simulink model "BatteryCtrl_V1"  (R2018a)
settings: Solver=VariableStepAuto  StartTime=0.0  StopTime=10.0  FixedStep=sampletime  RelTol=1e-3  EnableMultiTasking=on
PreLoadFcn:
  | BatteryCtrl_V1_BusInfo;
libraries: simulink x2
settings Model: Creator=IAEC nishito  LastModifiedBy=nishito
settings DataIOCC: LimitDataPoints=on  SaveFormat=Array  SignalLoggingSaveFormat=ModelDataLogs  SaveOutput=off
settings OptimizationCC: DefaultParameterBehavior=Inlined  ExpressionDepthLimit=2147483647  LifeSpan=inf
settings DebuggingCC: UnderspecifiedInitializationDetection=Classic  MergeDetectMultiDrivingBlocksExec=none  SolverPrmCheckMsg=warning  FcnCallInpInsideContextMsg=warning  StateNameClashWarn=warning  SFUnexpectedBacktrackingDiag=warning  SFNoUnconditionalDefaultTransitionDiag=warning  SFExecutionAtInitializationDiag=none
settings HardwareCC: ProdBitPerPointer=32  ProdBitPerSizeT=32  ProdBitPerPtrDiffT=32  ProdLargestAtomicFloat=None  ProdIntDivRoundTo=Undefined  ProdEndianess=Unspecified  ProdWordSize=32  ProdHWDeviceType=32-bit Generic
settings ModelReferenceCC: UpdateModelReferenceTargets=IfOutOfDate  PropagateSignalLabelsOutOfModel=off
settings CodeAppCC: StateflowObjectComments=on
settings GRTTargetCC: TargetLangStandard=C89/C90 (ANSI)  GeneratePreprocessorConditionals=Disable all  CombineOutputUpdateFcns=off  GRTInterface=on
settings ConfigComp: CovMetricSettings=dw  CovHtmlReporting=on  CovSaveCumulativeToWorkspaceVar=on  CovSaveSingleToWorkspaceVar=on  CovExternalEMLEnable=off  CovSFcnEnable=off

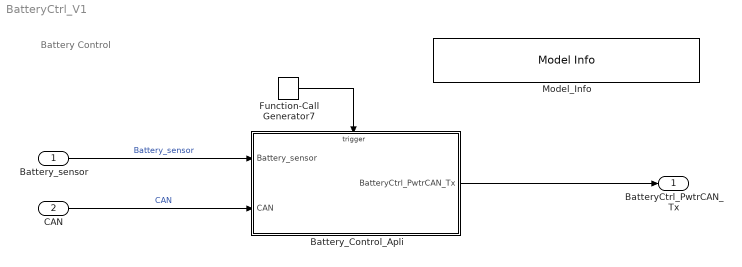
== system BatteryCtrl_V1 ==
  note: Battery Control
  Battery_sensor : Inport  OutDataTypeStr=Bus: Battery_sensor_Bus
      settings: AttributesFormatString=<%<OutDataTypeStr>>
  CAN : Inport  Port=2  OutDataTypeStr=Bus: CAN_Bus
      settings: AttributesFormatString=<%<OutDataTypeStr>>
  Battery_Control_Apli : Subsystem
  Function-Call Generator7 : simulink/Ports & Subsystems/Function-Call Generator  sample_time=0.05  numberOfIterations=1
      settings: AttributesFormatString=<sample_time=%<sample_time>>
  Model_Info : simulink/Model-Wide Utilities/Model Info  Frame=on  DisplayStringWithTags=|  HorizontalTextAlignment=Left  LeftAlignmentValue=0.02
      | Version  %<ModelVersion>
      | LastModifided by %<LastModifiedBy>  Date %<LastModificationDate>
      | Description  %<Description>
  BatteryCtrl_PwtrCAN_Tx : Outport  OutDataTypeStr=Bus: BatteryCtrl_PwtrCAN_Tx_Bus
      settings: AttributesFormatString=<%<OutDataTypeStr>>
  wires:
  Battery_Control_Apli/1(BatteryCtrl_PwtrCAN_Tx) -> BatteryCtrl_PwtrCAN_Tx/1
  CAN/1 -> Battery_Control_Apli/2(CAN)  "CAN"
  Battery_sensor/1 -> Battery_Control_Apli/1(Battery_sensor)  "Battery_sensor"
  Function-Call Generator7/1 -> Battery_Control_Apli/Trigger

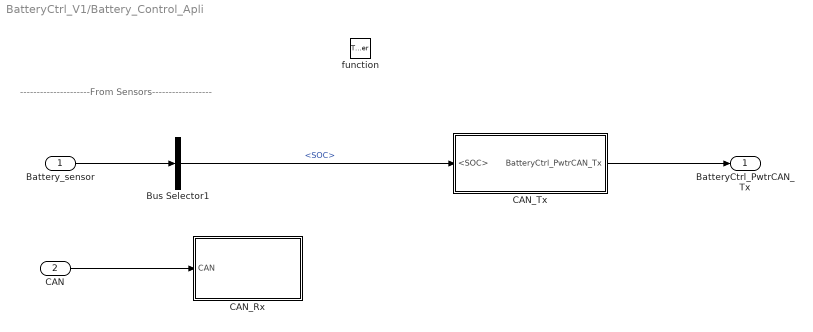
== system BatteryCtrl_V1/Battery_Control_Apli ==
  note: ---------------------From Sensors------------------
  Battery_sensor : Inport
  CAN : Inport  Port=2
  function : TriggerPort  TriggerType=function-call  VariantControl=Variant
  Bus Selector1 : BusSelector  OutputSignals=SOC
  CAN_Rx : Subsystem
  CAN_Tx : Subsystem
  BatteryCtrl_PwtrCAN_Tx : Outport
  wires:
  Battery_sensor/1 -> Bus Selector1/1
  Bus Selector1/1 -> CAN_Tx/1(<SOC>)  "<SOC>"
  CAN_Tx/1(BatteryCtrl_PwtrCAN_Tx) -> BatteryCtrl_PwtrCAN_Tx/1
  CAN/1 -> CAN_Rx/1(CAN)

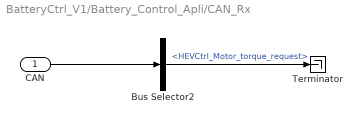
== system BatteryCtrl_V1/Battery_Control_Apli/CAN_Rx ==
  CAN : Inport
  Bus Selector2 : BusSelector  OutputSignals=PwtrCAN.HEV_Ctrl_PwtrCAN_Tx.HEVCtrl_Motor_torque_request
  Terminator : Terminator
  wires:
  CAN/1 -> Bus Selector2/1
  Bus Selector2/1 -> Terminator/1  "<HEVCtrl_Motor_torque_request>"

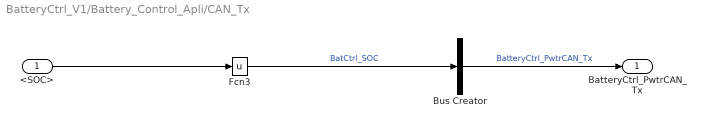
== system BatteryCtrl_V1/Battery_Control_Apli/CAN_Tx ==
  <SOC> : Inport
  Bus Creator : BusCreator  Inputs=1  OutDataTypeStr=Bus: BatteryCtrl_PwtrCAN_Tx_Bus
      settings: AttributesFormatString=<%<OutDataTypeStr>>
  Fcn3 : Fcn  Expr=u
  BatteryCtrl_PwtrCAN_Tx : Outport
  wires:
  Fcn3/1 -> Bus Creator/1  "BatCtrl_SOC"
  <SOC>/1 -> Fcn3/1
  Bus Creator/1 -> BatteryCtrl_PwtrCAN_Tx/1  "BatteryCtrl_PwtrCAN_Tx"
